simulink model "free_system"  (R2021b)
settings: Solver=VariableStepAuto  StartTime=0.0  StopTime=10.0  RelTol=1e-3
settings Model: Creator=lenna  LastModifiedBy=lenna

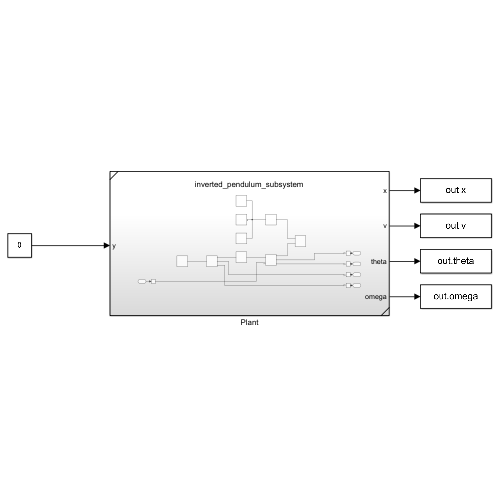
[thumbnail: Simulink's stored preview of the top-level diagram]
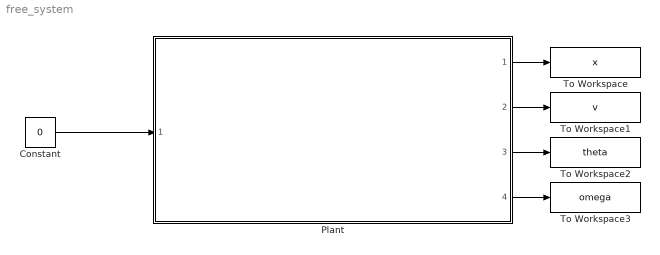
== system free_system ==
  Constant : Constant  Value=0
  Plant : Subsystem  ReferencedSubsystem=inverted_pendulum_subsystem
  To Workspace : ToWorkspace  VariableName=x  SaveFormat=Timeseries  SampleTime=-1
  To Workspace1 : ToWorkspace  VariableName=v  SaveFormat=Timeseries  SampleTime=-1
  To Workspace2 : ToWorkspace  VariableName=theta  SaveFormat=Timeseries  SampleTime=-1
  To Workspace3 : ToWorkspace  VariableName=omega  SaveFormat=Timeseries  SampleTime=-1
  wires:
  Constant/1 -> Plant/1
  Plant/1 -> To Workspace/1
  Plant/2 -> To Workspace1/1
  Plant/4 -> To Workspace3/1
  Plant/3 -> To Workspace2/1
